simulink model "RDEKF"  (R2020a)
settings: Solver=FixedStepAuto  StartTime=0.0  StopTime=t_sim  FixedStep=0.001  RelTol=1e-3
undefined symbols (not defined in the file or in its folder): initial_acceleration, initial_gyro, initial_orientation
libraries: vrlib x3, simulink x2
settings Model: Creator=addsd  LastModifiedBy=addsd
settings SFSimCC: CustomCodeUndefinedFunction=UseInterfaceOnly

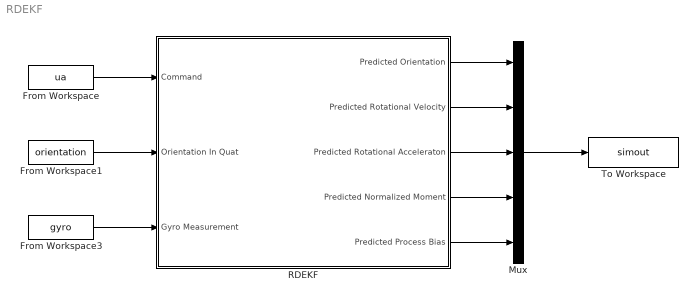
== system RDEKF ==
  From Workspace : FromWorkspace  VariableName=ua
  From Workspace1 : FromWorkspace  VariableName=orientation
  From Workspace3 : FromWorkspace  VariableName=gyro
  Mux : Mux  Inputs=[4 3 2 2 2]
  RDEKF : Subsystem  mask{q_init=initial_orientation, w_init=initial_gyro, o_init=initial_acceleration, P_init=eye(13), sig_gyro=[0.0019, 0.0056, 0.0001], sig_quat=[0.0001 0.0001 0.0001 0.0001], sig_u=[0.01 0.10]}
      mask prompts: q_init "Initial Orientation"; w_init "Initial Rotational Velocity"; o_init "Initial Rotational Acceleration"; P_init "Initial Covariance"; sig_gyro "Gyro Variance"; sig_quat "Orientation Measurement Variance"; sig_u "Process Variance"
      mask help:
      | DDTEKF For Qdrone 1234, dt set to 0.001, gravity vector set to [0 0 9.78909]
      | The Identified Parameters:
      | Kmz = 0.294861
      | Tmz = 0.017707
      | Td = [1.1629 1.1629 0.579374]
      mask init:
      | x_init = [q_init w_init o_init 0 0 0 0]';
      | 
      | Q = diag([sig_u]);
      | 
      | Q_tune = eye(13)*1e-6*0;
      | 
      | Q_tune(1:4, 1:4) = eye(4)*1e-6;
      | Q_tune(5:7, 5:7) = eye(3)*1e-3;
      | Q_tune(8:9, 8:9) = eye(2)*1e-4;
      | % Q_tune(10:11,10:11) = 1e-6;
      | % Q_tune(12:13,12:13) = 1e-6;
      | 
      | dHgyro = zeros(3, 13);
      | dHgyro(1:3, 5:7) = eye(3);
      | Rgyro = diag(sig_gyro).*eye(3);
      | 
      | dHquat = zeros(4, 13);
      | dHquat(1:4, 1:4) = eye(4);
      | Rquat = diag(sig_quat);
  To Workspace : ToWorkspace  VariableName=simout  SaveFormat=Timeseries  SampleTime=-1
  wires:
  Mux/1 -> To Workspace/1
  From Workspace/1 -> RDEKF/1(Command)
  RDEKF/1(Predicted Orientation) -> Mux/1
  RDEKF/2(Predicted Rotational Velocity) -> Mux/2
  RDEKF/3(Predicted Rotational Acceleraton) -> Mux/3
  RDEKF/4(Predicted Normalized Moment) -> Mux/4
  RDEKF/5(Predicted Process Bias) -> Mux/5
  From Workspace3/1 -> RDEKF/3(Gyro Measurement)
  From Workspace1/1 -> RDEKF/2(Orientation In Quat)

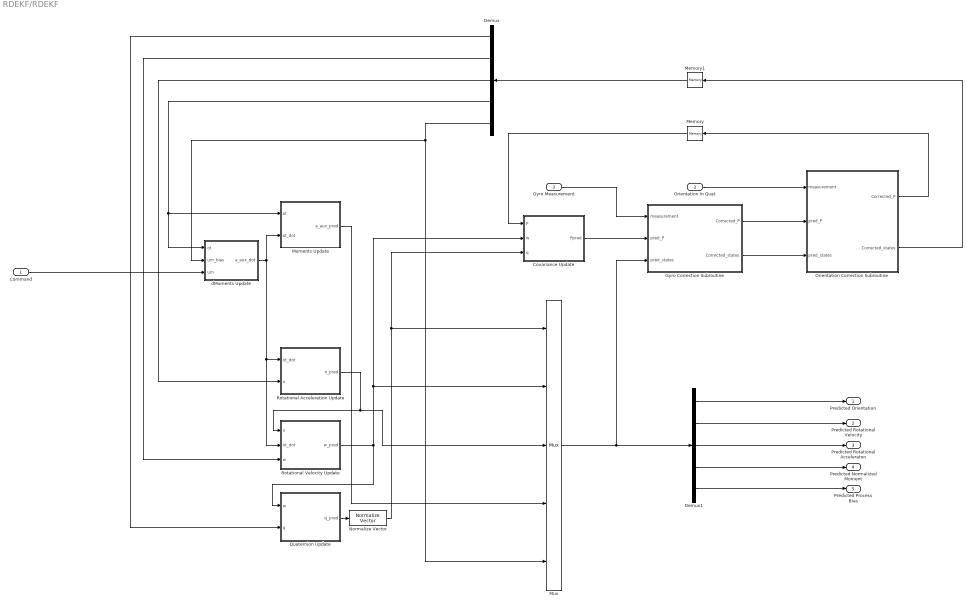
== system RDEKF/RDEKF ==
  Command : Inport
  Orientation In Quat : Inport  Port=2
  Gyro Measurement : Inport  Port=3
  Covariance Update : Subsystem
  Demux : Demux  Outputs=[4 3 2 2 2]
  Demux1 : Demux  Outputs=[4 3 2 2 2]
  Gyro Correction Subroutine : Subsystem
  Memory : Memory  InitialCondition=P_init
  Memory1 : Memory  InitialCondition=x_init
  Moments Update : Subsystem
  Mux : Mux  Inputs=[4 3 2 2 2]
  Normalize Vector : vrlib/Utilities/Normalize Vector  maxzero=0
  Orientation Correction Subroutine : Subsystem  TreatAsAtomicUnit=on
  Quaternion Update : Subsystem
  Rotational Acceleration Update : Subsystem
  Rotational Velocity Update : Subsystem
  dMoments Update : Subsystem
  Predicted Orientation : Outport
  Predicted Rotational Velocity : Outport  Port=2
  Predicted Rotational Acceleraton : Outport  Port=3
  Predicted Normalized Moment : Outport  Port=4
  Predicted Process Bias : Outport  Port=5
  wires:
  dMoments Update/1(a_aux_dot) -> Moments Update/2(ot_dot), Rotational Velocity Update/2(ot_dot), Rotational Acceleration Update/1(ot_dot)
  Command/1 -> dMoments Update/3(um)
  Demux/4 -> Moments Update/1(ot), dMoments Update/1(ot)
  Rotational Acceleration Update/1(o_pred) -> Mux/3, Rotational Velocity Update/1(o)
  Rotational Velocity Update/1(w_pred) -> Quaternion Update/1(w), Mux/2, Covariance Update/2(w)
  Moments Update/1(a_aux_pred) -> Mux/4
  Mux/1 -> Demux1/1, Gyro Correction Subroutine/3(pred_states)
  Gyro Correction Subroutine/1(Corrected_P) -> Orientation Correction Subroutine/2("pred_P ")
  Memory/1 -> Covariance Update/1(P)
  Memory1/1 -> Demux/1
  Demux1/2 -> Predicted Rotational Velocity/1
  Demux1/1 -> Predicted Orientation/1
  Demux1/3 -> Predicted Rotational Acceleraton/1
  Demux1/5 -> Predicted Process Bias/1
  Demux1/4 -> Predicted Normalized Moment/1
  Gyro Measurement/1 -> Gyro Correction Subroutine/1(measurement)
  Orientation In Quat/1 -> Orientation Correction Subroutine/1(measurement)
  Demux/1 -> Quaternion Update/2(q)
  Demux/3 -> Rotational Acceleration Update/2(o)
  Demux/2 -> Rotational Velocity Update/3(w)
  Quaternion Update/1(q_pred) -> Normalize Vector/1
  Covariance Update/1(Ppred) -> Gyro Correction Subroutine/2("pred_P ")
  Orientation Correction Subroutine/1(Corrected_P) -> Memory/1
  Normalize Vector/1 -> Mux/1, Covariance Update/3(q)
  Gyro Correction Subroutine/2(Corrected_states) -> Orientation Correction Subroutine/3(pred_states)
  Orientation Correction Subroutine/2(Corrected_states) -> Memory1/1
  Demux/5 -> dMoments Update/2(um_bias), Mux/5

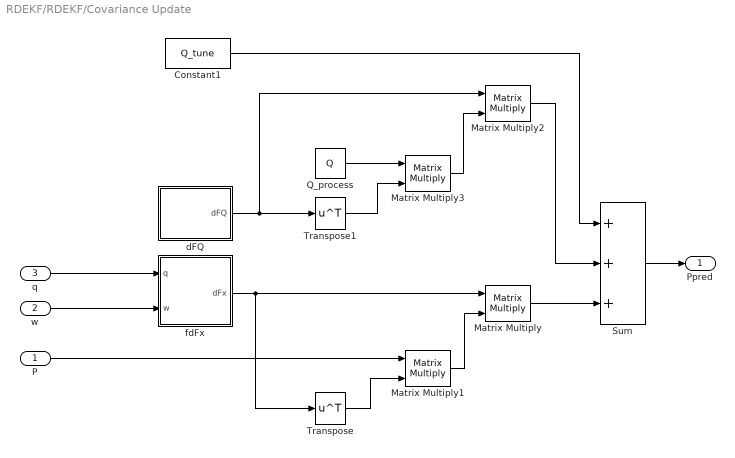
== system RDEKF/RDEKF/Covariance Update ==
  P : Inport
  w : Inport  Port=2
  q : Inport  Port=3
  Constant1 : Constant  Value=Q_tune
  Matrix Multiply{,1..3} (4 alike) : Product  Multiplication=Matrix(*)
  Q_process : Constant  Value=Q
  Sum : Sum  Inputs=+++
  Transpose : Math  Operator=transpose  SaturateOnIntegerOverflow=on
  Transpose1 : Math  Operator=transpose  SaturateOnIntegerOverflow=on
  dFQ : MATLAB Function  TreatAsAtomicUnit=on
  fdFx : MATLAB Function  TreatAsAtomicUnit=on
  Ppred : Outport
  wires:
  Matrix Multiply3/1 -> Matrix Multiply2/2
  Transpose1/1 -> Matrix Multiply3/2
  Matrix Multiply1/1 -> Matrix Multiply/2
  fdFx/1(dFx) -> Transpose/1, Matrix Multiply/1
  Transpose/1 -> Matrix Multiply1/2
  Q_process/1 -> Matrix Multiply3/1
  dFQ/1(dFQ) -> Matrix Multiply2/1, Transpose1/1
  Matrix Multiply2/1 -> Sum/2
  Matrix Multiply/1 -> Sum/3
  Sum/1 -> Ppred/1
  Constant1/1 -> Sum/1
  q/1 -> fdFx/1(q)
  P/1 -> Matrix Multiply1/1
  w/1 -> fdFx/2(w)

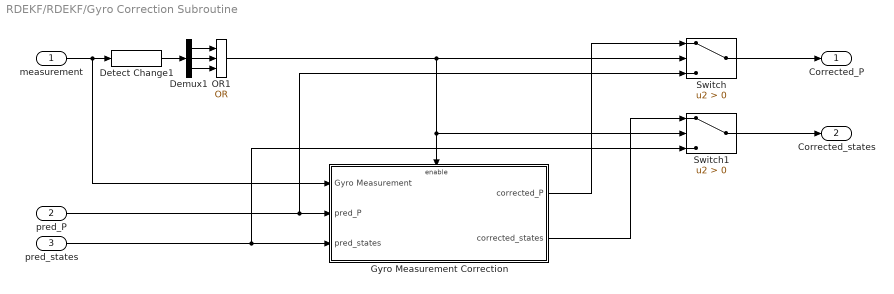
== system RDEKF/RDEKF/Gyro Correction Subroutine ==
  measurement : Inport
  "pred_P " : Inport  Port=2
  pred_states : Inport  Port=3
  Demux1 : Demux  Outputs=3
  Detect Change1 : simulink/Logic and Bit Operations/Detect Change  vinit=[0;0;0]  OutDataTypeStr=boolean
  Gyro Measurement Correction : Subsystem
  OR1 : Logic  Operator=OR  Inputs=3  IconShape=distinctive  AllPortsSameDT=off  OutDataTypeStr=boolean
  Switch : Switch  Criteria=u2 > Threshold
  Switch1 : Switch  Criteria=u2 > Threshold
  Corrected_P : Outport
  Corrected_states : Outport  Port=2
  wires:
  Demux1/1 -> OR1/1
  measurement/1 -> Gyro Measurement Correction/1(Gyro Measurement), Detect Change1/1
  Demux1/3 -> OR1/3
  OR1/1 -> Gyro Measurement Correction/Enable, Switch1/2, Switch/2
  Detect Change1/1 -> Demux1/1
  Demux1/2 -> OR1/2
  Switch1/1 -> Corrected_states/1
  "pred_P "/1 -> Switch/3, Gyro Measurement Correction/2("pred_P ")
  pred_states/1 -> Switch1/3, Gyro Measurement Correction/3(pred_states)
  Gyro Measurement Correction/2(corrected_states) -> Switch1/1
  Switch/1 -> Corrected_P/1
  Gyro Measurement Correction/1(corrected_P) -> Switch/1

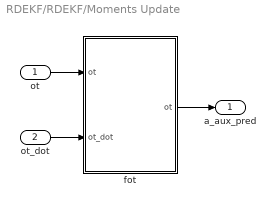
== system RDEKF/RDEKF/Moments Update ==
  ot : Inport
  ot_dot : Inport  Port=2
  fot : MATLAB Function  TreatAsAtomicUnit=on
  a_aux_pred : Outport
  wires:
  ot/1 -> fot/1("ot ")
  ot_dot/1 -> fot/2(ot_dot)
  fot/1(ot) -> a_aux_pred/1

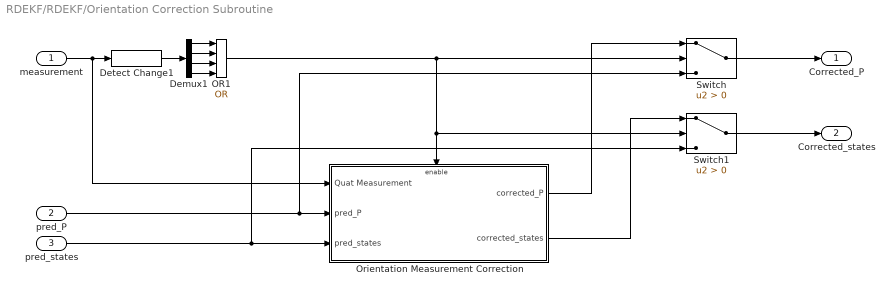
== system RDEKF/RDEKF/Orientation Correction Subroutine ==
  measurement : Inport
  "pred_P " : Inport  Port=2
  pred_states : Inport  Port=3
  Demux1 : Demux
  Detect Change1 : simulink/Logic and Bit Operations/Detect Change  vinit=[1;0;0;0]  OutDataTypeStr=boolean
  OR1 : Logic  Operator=OR  Inputs=4  IconShape=distinctive  AllPortsSameDT=off  OutDataTypeStr=boolean
  Orientation Measurement Correction : Subsystem
  Switch : Switch  Criteria=u2 > Threshold
  Switch1 : Switch  Criteria=u2 > Threshold
  Corrected_P : Outport
  Corrected_states : Outport  Port=2
  wires:
  Demux1/1 -> OR1/1
  measurement/1 -> Orientation Measurement Correction/1(Quat Measurement), Detect Change1/1
  Demux1/3 -> OR1/3
  Detect Change1/1 -> Demux1/1
  Demux1/2 -> OR1/2
  Switch1/1 -> Corrected_states/1
  "pred_P "/1 -> Orientation Measurement Correction/2("pred_P "), Switch/3
  pred_states/1 -> Orientation Measurement Correction/3(pred_states), Switch1/3
  Orientation Measurement Correction/2(corrected_states) -> Switch1/1
  Switch/1 -> Corrected_P/1
  Orientation Measurement Correction/1(corrected_P) -> Switch/1
  OR1/1 -> Switch1/2, Orientation Measurement Correction/Enable, Switch/2
  Demux1/4 -> OR1/4

== system RDEKF/RDEKF/Quaternion Update ==
  w : Inport
  q : Inport  Port=2
  fq : MATLAB Function  TreatAsAtomicUnit=on
  q_pred : Outport
  wires:
  fq/1(fq) -> q_pred/1
  w/1 -> fq/2(w)
  q/1 -> fq/1(q)

== system RDEKF/RDEKF/Rotational Acceleration Update ==
  ot_dot : Inport
  o : Inport  Port=2
  fo : MATLAB Function  TreatAsAtomicUnit=on
  o_pred : Outport
  wires:
  fo/1(fo) -> o_pred/1
  ot_dot/1 -> fo/1(ot_dot)
  o/1 -> fo/2(o)

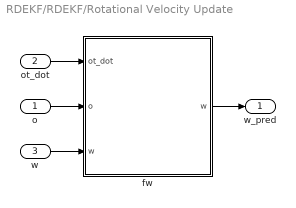
== system RDEKF/RDEKF/Rotational Velocity Update ==
  o : Inport
  ot_dot : Inport  Port=2
  w : Inport  Port=3
  fw : MATLAB Function  TreatAsAtomicUnit=on
  w_pred : Outport
  wires:
  fw/1(w) -> w_pred/1
  ot_dot/1 -> fw/1(ot_dot)
  o/1 -> fw/2(o)
  w/1 -> fw/3("w ")

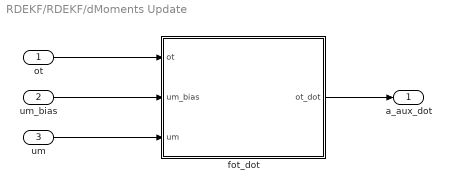
== system RDEKF/RDEKF/dMoments Update ==
  ot : Inport
  um_bias : Inport  Port=2
  um : Inport  Port=3
  fot_dot : MATLAB Function  TreatAsAtomicUnit=on
  a_aux_dot : Outport
  wires:
  fot_dot/1(ot_dot) -> a_aux_dot/1
  ot/1 -> fot_dot/1(ot)
  um/1 -> fot_dot/3(um)
  um_bias/1 -> fot_dot/2(um_bias)

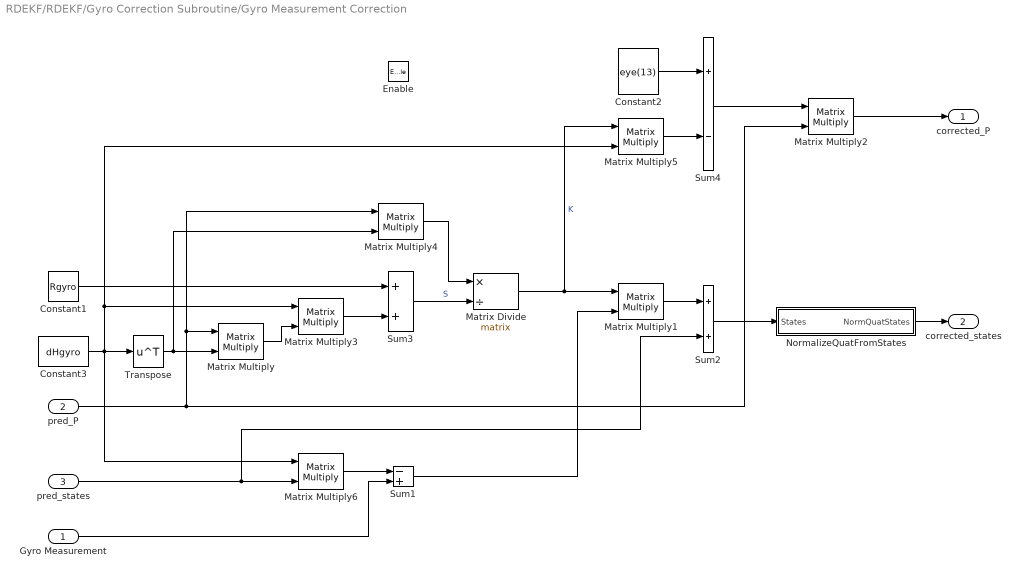
== system RDEKF/RDEKF/Gyro Correction Subroutine/Gyro Measurement Correction ==
  Gyro Measurement : Inport
  "pred_P " : Inport  Port=2
  pred_states : Inport  Port=3
  Enable : EnablePort
  Constant1 : Constant  Value=Rgyro
  Constant2 : Constant  Value=eye(13)
  Constant3 : Constant  Value=dHgyro  VectorParams1D=off
  Matrix Divide : Product  Inputs=*/  Multiplication=Matrix(*)
  Matrix Multiply{,1..6} (7 alike) : Product  Multiplication=Matrix(*)
  NormalizeQuatFromStates : Subsystem
  Sum1 : Sum  Inputs=-+
  Sum2 : Sum
  Sum3 : Sum
  Sum4 : Sum  Inputs=+-
  Transpose : Math  Operator=transpose  SaturateOnIntegerOverflow=on
  corrected_P : Outport
  corrected_states : Outport  Port=2
  wires:
  Constant3/1 -> Matrix Multiply6/1, Matrix Multiply5/2, Matrix Multiply3/1, Transpose/1
  Matrix Multiply4/1 -> Matrix Divide/1
  Sum3/1 -> Matrix Divide/2  "S"
  Matrix Multiply/1 -> Matrix Multiply3/2
  Matrix Multiply3/1 -> Sum3/2
  Transpose/1 -> Matrix Multiply4/2, Matrix Multiply/2
  Constant1/1 -> Sum3/1
  Matrix Multiply6/1 -> Sum1/1
  Gyro Measurement/1 -> Sum1/2
  pred_states/1 -> Sum2/2, Matrix Multiply6/2
  Matrix Divide/1 -> Matrix Multiply5/1, Matrix Multiply1/1  "K"
  Sum1/1 -> Matrix Multiply1/2
  Matrix Multiply1/1 -> Sum2/1
  Sum2/1 -> NormalizeQuatFromStates/1(States)
  Matrix Multiply5/1 -> Sum4/2
  Sum4/1 -> Matrix Multiply2/1
  Constant2/1 -> Sum4/1
  Matrix Multiply2/1 -> corrected_P/1
  "pred_P "/1 -> Matrix Multiply2/2, Matrix Multiply4/1, Matrix Multiply/1
  NormalizeQuatFromStates/1(NormQuatStates) -> corrected_states/1

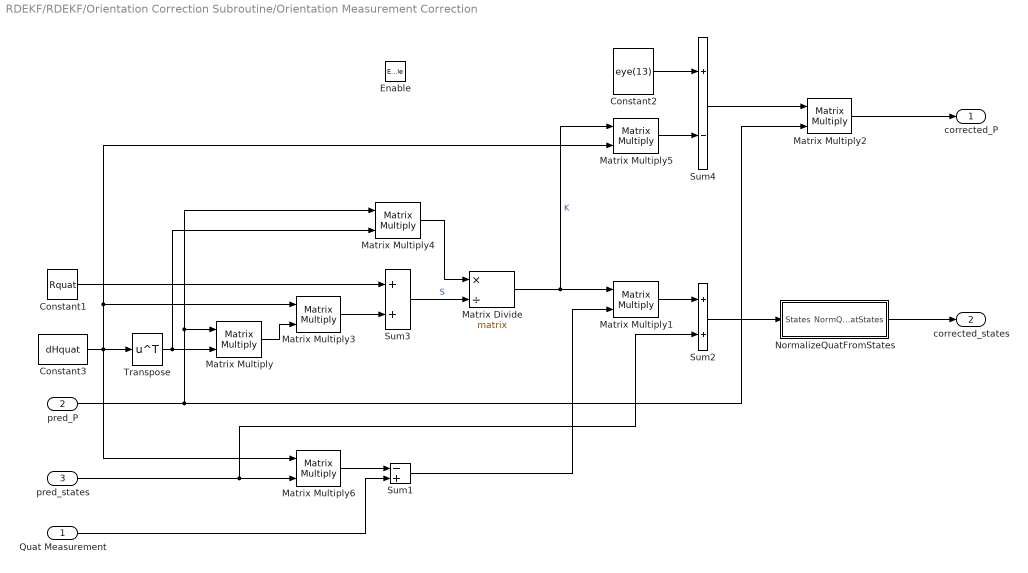
== system RDEKF/RDEKF/Orientation Correction Subroutine/Orientation Measurement Correction ==
  Quat Measurement : Inport
  "pred_P " : Inport  Port=2
  pred_states : Inport  Port=3
  Enable : EnablePort
  Constant1 : Constant  Value=Rquat
  Constant2 : Constant  Value=eye(13)
  Constant3 : Constant  Value=dHquat  VectorParams1D=off
  Matrix Divide : Product  Inputs=*/  Multiplication=Matrix(*)
  Matrix Multiply{,1..6} (7 alike) : Product  Multiplication=Matrix(*)
  NormalizeQuatFromStates : Subsystem
  Sum1 : Sum  Inputs=-+
  Sum2 : Sum
  Sum3 : Sum
  Sum4 : Sum  Inputs=+-
  Transpose : Math  Operator=transpose  SaturateOnIntegerOverflow=on
  corrected_P : Outport
  corrected_states : Outport  Port=2
  wires:
  Constant3/1 -> Matrix Multiply6/1, Matrix Multiply5/2, Matrix Multiply3/1, Transpose/1
  Matrix Multiply4/1 -> Matrix Divide/1
  Sum3/1 -> Matrix Divide/2  "S"
  Matrix Multiply/1 -> Matrix Multiply3/2
  Matrix Multiply3/1 -> Sum3/2
  Transpose/1 -> Matrix Multiply4/2, Matrix Multiply/2
  Constant1/1 -> Sum3/1
  Matrix Multiply6/1 -> Sum1/1
  Quat Measurement/1 -> Sum1/2
  pred_states/1 -> Sum2/2, Matrix Multiply6/2
  Matrix Divide/1 -> Matrix Multiply5/1, Matrix Multiply1/1  "K"
  Sum1/1 -> Matrix Multiply1/2
  Matrix Multiply1/1 -> Sum2/1
  Sum2/1 -> NormalizeQuatFromStates/1(States)
  Matrix Multiply5/1 -> Sum4/2
  Sum4/1 -> Matrix Multiply2/1
  Constant2/1 -> Sum4/1
  Matrix Multiply2/1 -> corrected_P/1
  "pred_P "/1 -> Matrix Multiply2/2, Matrix Multiply4/1, Matrix Multiply/1
  NormalizeQuatFromStates/1(NormQuatStates) -> corrected_states/1

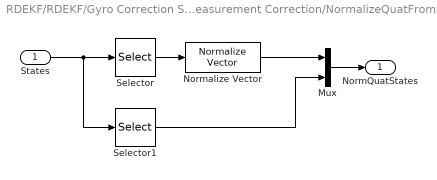
== system RDEKF/RDEKF/Gyro Correction Subroutine/Gyro Measurement Correction/NormalizeQuatFromStates ==
  States : Inport
  Mux : Mux  Inputs=[4 9]
  Normalize Vector : vrlib/Utilities/Normalize Vector  maxzero=0
  Selector : Selector  InputPortWidth=13  IndexOptions=Index vector (dialog)  Indices=[1:4]  OutputSizes=1
  Selector1 : Selector  InputPortWidth=13  IndexOptions=Index vector (dialog)  Indices=[5:13]  OutputSizes=1
  NormQuatStates : Outport
  wires:
  States/1 -> Selector1/1, Selector/1
  Selector/1 -> Normalize Vector/1
  Selector1/1 -> Mux/2
  Mux/1 -> NormQuatStates/1
  Normalize Vector/1 -> Mux/1

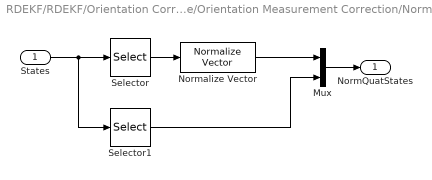
== system RDEKF/RDEKF/Orientation Correction Subroutine/Orientation Measurement Correction/NormalizeQuatFromStates ==
  States : Inport
  Mux : Mux  Inputs=[4 9]
  Normalize Vector : vrlib/Utilities/Normalize Vector  maxzero=0
  Selector : Selector  InputPortWidth=13  IndexOptions=Index vector (dialog)  Indices=[1:4]  OutputSizes=1
  Selector1 : Selector  InputPortWidth=13  IndexOptions=Index vector (dialog)  Indices=[5:13]  OutputSizes=1
  NormQuatStates : Outport
  wires:
  States/1 -> Selector1/1, Selector/1
  Selector/1 -> Normalize Vector/1
  Selector1/1 -> Mux/2
  Mux/1 -> NormQuatStates/1
  Normalize Vector/1 -> Mux/1

== matlab function RDEKF/Covariance Update/dFQ ==
  data: dFQ output
function dFQ = fdFQ
%FDFQA
%    DFQA = FDFQA

%    This function was generated by the Symbolic Math Toolbox version 8.5.
%    25-May-2021 19:36:20

dFQ = reshape([0.0,0.0,0.0,0.0,2.275630262630313e-3,0.0,0.0,4.551260525260625,0.0,4.551260525260625,0.0,0.0,0.0,0.0,0.0,0.0,0.0,0.0,2.375889635124298e-3,0.0,0.0,4.751779270248597,0.0,4.751779270248597,0.0,0.0],[13,2]);

== matlab function RDEKF/Covariance Update/fdFx ==
  data: q input; dFx output; w input
function dFx = fdFx(q, w)
%FDFXA
%    DFXA = FDFXA(q(1),q(2),q(3),q(4),w(1),w(2),w(3))

%    This function was generated by the Symbolic Math Toolbox version 8.5.
%    25-May-2021 19:35:08

t2 = q(1)./2.0e+3;
t3 = q(2)./2.0e+3;
t4 = q(3)./2.0e+3;
t5 = q(4)./2.0e+3;
t6 = w(1)./2.0e+3;
t7 = w(2)./2.0e+3;
t8 = w(3)./2.0e+3;
t9 = -t3;
t10 = -t4;
t11 = -t5;
t12 = -t6;
t13 = -t7;
t14 = -t8;
dFx = reshape([1.0,t6,t7,t8,0.0,0.0,0.0,0.0,0.0,0.0,0.0,0.0,0.0,t12,1.0,t14,t7,0.0,0.0,0.0,0.0,0.0,0.0,0.0,0.0,0.0,t13,t8,1.0,t12,0.0,0.0,0.0,0.0,0.0,0.0,0.0,0.0,0.0,t14,t13,t6,1.0,0.0,0.0,0.0,0.0,0.0,0.0,0.0,0.0,0.0,t9,t2,t5,t10,1.0,0.0,0.0,0.0,0.0,0.0,0.0,0.0,0.0,t10,t11,t2,t3,0.0,1.0,0.0,0.0,0.0,0.0,0.0,0.0,0.0,t11,t4,t9,t2,0.0,0.0,1.0,0.0,0.0,0.0,0.0,0.0,0.0,0.0,0.0,0.0,0.0,9.979951884522855e-4,0.0,0.0,9.95990376904571e-1,0.0,0.0,0.0,0.0,0.0,0.0,0.0,0.0,0.0,0.0,9.979951884522855e-4,0.0,0.0,9.95990376904571e-1,0.0,0.0,0.0,0.0,0.0,0.0,0.0,0.0,-7.8125e-6,0.0,0.0,-1.0./6.4e+1,0.0,6.3e+1./6.4e+1,0.0,0.0,0.0,0.0,0.0,0.0,0.0,0.0,-7.8125e-6,0.0,0.0,-1.0./6.4e+1,0.0,6.3e+1./6.4e+1,0.0,0.0,0.0,0.0,0.0,0.0,-2.275630262630313e-3,0.0,0.0,-4.551260525260625,0.0,-4.551260525260625,0.0,1.0,0.0,0.0,0.0,0.0,0.0,0.0,-2.375889635124298e-3,0.0,0.0,-4.751779270248597,0.0,-4.751779270248597,0.0,1.0],[13,13]);

== matlab function RDEKF/Rotational Acceleration Update/fo ==
  data: ot_dot input; fo output; o input
function fo = fo(ot_dot, o)
%FO
%    FO = FO(a_aux_dot(1),a_aux_dot(2),o(1),o(2))

%    This function was generated by the Symbolic Math Toolbox version 8.5.
%    25-May-2021 19:40:00

fo = [ot_dot(1)./1.0e+3+o(1).*9.95990376904571e-1;ot_dot(2)./1.0e+3+o(2).*9.95990376904571e-1];

== matlab function RDEKF/Rotational Velocity Update/fw ==
  data: ot_dot input; w output; o input; w input
function w = fw(ot_dot, o, w)
%FW
%    FW = FW(a_aux_dot(1),a_aux_dot(2),o(1),o(2),w(1),w(2),w(3))

%    This function was generated by the Symbolic Math Toolbox version 8.5.
%    25-May-2021 19:40:57

w = [ot_dot(1)./2.0e+6+o(1).*9.979951884522855e-4+w(1);ot_dot(2)./2.0e+6+o(2).*9.979951884522855e-4+w(2);w(3)];

== matlab function RDEKF/Quaternion Update/fq ==
  data: q input; w input; fq output
function fq = fq(q, w)
%FQ
%    FQ = FQ(Q1,Q2,Q3,Q4,W1,W2,W3)

%    This function was generated by the Symbolic Math Toolbox version 8.5.
%    15-Apr-2021 09:35:16

fq = [q(1)-(q(2).*w(1))./2.0e+3-(q(3).*w(2))./2.0e+3-(q(4).*w(3))./2.0e+3;q(2)+(q(1).*w(1))./2.0e+3+(q(3).*w(3))./2.0e+3-(q(4).*w(2))./2.0e+3;q(3)+(q(1).*w(2))./2.0e+3-(q(2).*w(3))./2.0e+3+(q(4).*w(1))./2.0e+3;q(4)+(q(1).*w(3))./2.0e+3+(q(2).*w(2))./2.0e+3-(q(3).*w(1))./2.0e+3];

== matlab function RDEKF/dMoments Update/fot_dot ==
  data: ot input; ot_dot output; um_bias input; um input
function ot_dot = fot_dot(ot, um_bias, um)
%FA_AUX_DOT
%    FA_AUX_DOT = FA_AUX_DOT(a_aux(1),a_aux(2),a_aux_b(1),a_aux_b(2),ua(1),ua(2))

%    This function was generated by the Symbolic Math Toolbox version 8.5.
%    25-May-2021 19:37:06

ot_dot = [ot(1).*(-1.25e+2./8.0)-um_bias(1).*4.551260525260625e+3+um(1).*4.551260525260625e+3;ot(2).*(-1.25e+2./8.0)-um_bias(2).*4.751779270248597e+3+um(2).*4.751779270248597e+3];

== matlab function RDEKF/Moments Update/fot ==
  data: ot input; ot output; ot_dot input
function ot = fot(ot, ot_dot)
%FA_AUX
%    FA_AUX = FA_AUX(a_aux(1),a_aux(2),a_aux_dot(1),a_aux_dot(2))

%    This function was generated by the Symbolic Math Toolbox version 8.5.
%    25-May-2021 19:39:01

ot = [ot(1)+ot_dot(1)./1.0e+3;ot(2)+ot_dot(2)./1.0e+3];
